simulink model "Modelo_UAV"  (R2017b)
settings: Solver=FixedStepAuto  StartTime=0.0  StopTime=6  FixedStep=1/10000  RelTol=1e-3
values from neighbouring files (symbols this model uses):
  Jcm_x = 7.5e3    (= 7500)    [UAV_parametros.m]
  Jcm_y = 7.5e3    (= 7500)    [UAV_parametros.m]
  Jcm_z = 14e3    (= 14000)    [UAV_parametros.m]
  M_t = 0.6    [UAV_parametros.m]
undefined symbols (not defined in the file or in its folder): sigbuilder_block
libraries: simulink x4
settings Model: Creator=JUANSEBASTIAN  LastModifiedBy=JUANSEBASTIAN
settings OptimizationCC: LifeSpan=inf
settings DebuggingCC: SFExecutionAtInitializationDiag=none
settings CodeAppCC: StateflowObjectComments=on

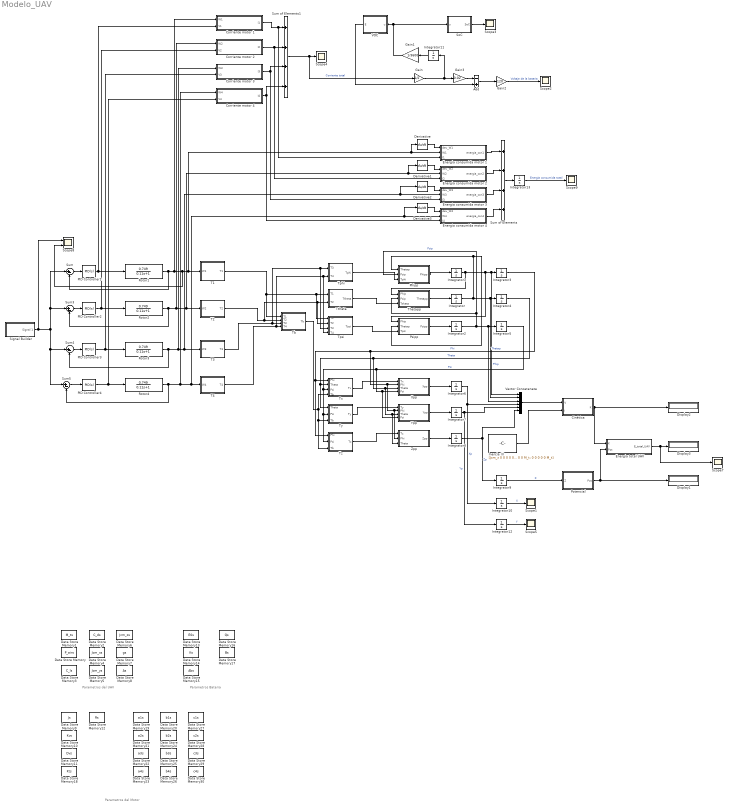
== system Modelo_UAV ==
  note: Parametros del UAV
  note: Parametros del Motor
  note: Parametros Bateria
  Add : Sum  Inputs=-+
  Cinética : MATLAB Function  TreatAsAtomicUnit=on
  Corriente motor 1 : MATLAB Function  TreatAsAtomicUnit=on
  Corriente motor 2 : MATLAB Function  TreatAsAtomicUnit=on
  Corriente motor 3 : MATLAB Function  TreatAsAtomicUnit=on
  Corriente motor 4 : MATLAB Function  TreatAsAtomicUnit=on
  Data Store Memory : DataStoreMemory  DataStoreName=P_airs  ReadBeforeWriteMsg=warning  WriteAfterWriteMsg=warning  WriteAfterReadMsg=warning  InitialValue=P_air  ShowAdditionalParam=off  OutDataTypeStr=double
      settings: LockScale=on
  Data Store Memory1 : DataStoreMemory  DataStoreName=M_ts  ReadBeforeWriteMsg=warning  WriteAfterWriteMsg=warning  WriteAfterReadMsg=warning  InitialValue=M_t  ShowAdditionalParam=off  OutDataTypeStr=double
      settings: LockScale=on
  Data Store Memory10 : DataStoreMemory  DataStoreName=Kvs  ReadBeforeWriteMsg=warning  WriteAfterWriteMsg=warning  WriteAfterReadMsg=warning  InitialValue=Kv  ShowAdditionalParam=off  OutDataTypeStr=double
      settings: LockScale=on
  Data Store Memory11 : DataStoreMemory  DataStoreName=Dvs  ReadBeforeWriteMsg=warning  WriteAfterWriteMsg=warning  WriteAfterReadMsg=warning  InitialValue=Dv  ShowAdditionalParam=off  OutDataTypeStr=double
      settings: LockScale=on
  Data Store Memory12 : DataStoreMemory  DataStoreName=Rs  ReadBeforeWriteMsg=warning  WriteAfterWriteMsg=warning  WriteAfterReadMsg=warning  InitialValue=R  ShowAdditionalParam=off  OutDataTypeStr=double
      settings: LockScale=on
  Data Store Memory13 : DataStoreMemory  DataStoreName=E0s  ReadBeforeWriteMsg=warning  WriteAfterWriteMsg=warning  WriteAfterReadMsg=warning  InitialValue=E0  ShowAdditionalParam=off  OutDataTypeStr=double
      settings: LockScale=on
  Data Store Memory14 : DataStoreMemory  DataStoreName=Ks  ReadBeforeWriteMsg=warning  WriteAfterWriteMsg=warning  WriteAfterReadMsg=warning  InitialValue=K  ShowAdditionalParam=off  OutDataTypeStr=double
      settings: LockScale=on
  Data Store Memory15 : DataStoreMemory  DataStoreName=Abs  ReadBeforeWriteMsg=warning  WriteAfterWriteMsg=warning  WriteAfterReadMsg=warning  InitialValue=Ab  ShowAdditionalParam=off  OutDataTypeStr=double
      settings: LockScale=on
  Data Store Memory16 : DataStoreMemory  DataStoreName=Qs  ReadBeforeWriteMsg=warning  WriteAfterWriteMsg=warning  WriteAfterReadMsg=warning  InitialValue=Q  ShowAdditionalParam=off  OutDataTypeStr=double
      settings: LockScale=on
  Data Store Memory17 : DataStoreMemory  DataStoreName=Bs  ReadBeforeWriteMsg=warning  WriteAfterWriteMsg=warning  WriteAfterReadMsg=warning  InitialValue=B  ShowAdditionalParam=off  OutDataTypeStr=double
      settings: LockScale=on
  Data Store Memory18 : DataStoreMemory  DataStoreName=Kts  ReadBeforeWriteMsg=warning  WriteAfterWriteMsg=warning  WriteAfterReadMsg=warning  InitialValue=Kt  ShowAdditionalParam=off  OutDataTypeStr=double
      settings: LockScale=on
  Data Store Memory19 : DataStoreMemory  DataStoreName=a1s  ReadBeforeWriteMsg=warning  WriteAfterWriteMsg=warning  WriteAfterReadMsg=warning  InitialValue=a1  ShowAdditionalParam=off  OutDataTypeStr=double
      settings: LockScale=on
  Data Store Memory2 : DataStoreMemory  DataStoreName=C_ds  ReadBeforeWriteMsg=warning  WriteAfterWriteMsg=warning  WriteAfterReadMsg=warning  InitialValue=C_d  ShowAdditionalParam=off  OutDataTypeStr=double
      settings: LockScale=on
  Data Store Memory20 : DataStoreMemory  DataStoreName=b1s  ReadBeforeWriteMsg=warning  WriteAfterWriteMsg=warning  WriteAfterReadMsg=warning  InitialValue=b1  ShowAdditionalParam=off  OutDataTypeStr=double
      settings: LockScale=on
  Data Store Memory21 : DataStoreMemory  DataStoreName=a2s  ReadBeforeWriteMsg=warning  WriteAfterWriteMsg=warning  WriteAfterReadMsg=warning  InitialValue=a2  ShowAdditionalParam=off  OutDataTypeStr=double
      settings: LockScale=on
  Data Store Memory22 : DataStoreMemory  DataStoreName=a3s  ReadBeforeWriteMsg=warning  WriteAfterWriteMsg=warning  WriteAfterReadMsg=warning  InitialValue=a3  ShowAdditionalParam=off  OutDataTypeStr=double
      settings: LockScale=on
  Data Store Memory23 : DataStoreMemory  DataStoreName=a4s  ReadBeforeWriteMsg=warning  WriteAfterWriteMsg=warning  WriteAfterReadMsg=warning  InitialValue=a4  ShowAdditionalParam=off  OutDataTypeStr=double
      settings: LockScale=on
  Data Store Memory24 : DataStoreMemory  DataStoreName=b2s  ReadBeforeWriteMsg=warning  WriteAfterWriteMsg=warning  WriteAfterReadMsg=warning  InitialValue=b2  ShowAdditionalParam=off  OutDataTypeStr=double
      settings: LockScale=on
  Data Store Memory25 : DataStoreMemory  DataStoreName=b3s  ReadBeforeWriteMsg=warning  WriteAfterWriteMsg=warning  WriteAfterReadMsg=warning  InitialValue=b3  ShowAdditionalParam=off  OutDataTypeStr=double
      settings: LockScale=on
  Data Store Memory26 : DataStoreMemory  DataStoreName=b4s  ReadBeforeWriteMsg=warning  WriteAfterWriteMsg=warning  WriteAfterReadMsg=warning  InitialValue=b4  ShowAdditionalParam=off  OutDataTypeStr=double
      settings: LockScale=on
  Data Store Memory27 : DataStoreMemory  DataStoreName=c1s  ReadBeforeWriteMsg=warning  WriteAfterWriteMsg=warning  WriteAfterReadMsg=warning  InitialValue=c1  ShowAdditionalParam=off  OutDataTypeStr=double
      settings: LockScale=on
  Data Store Memory28 : DataStoreMemory  DataStoreName=c2s  ReadBeforeWriteMsg=warning  WriteAfterWriteMsg=warning  WriteAfterReadMsg=warning  InitialValue=c2  ShowAdditionalParam=off  OutDataTypeStr=double
      settings: LockScale=on
  Data Store Memory29 : DataStoreMemory  DataStoreName=c3s  ReadBeforeWriteMsg=warning  WriteAfterWriteMsg=warning  WriteAfterReadMsg=warning  InitialValue=c3  ShowAdditionalParam=off  OutDataTypeStr=double
      settings: LockScale=on
  Data Store Memory3 : DataStoreMemory  DataStoreName=C_ls  ReadBeforeWriteMsg=warning  WriteAfterWriteMsg=warning  WriteAfterReadMsg=warning  InitialValue=C_l  ShowAdditionalParam=off  OutDataTypeStr=double
      settings: LockScale=on
  Data Store Memory30 : DataStoreMemory  DataStoreName=c4s  ReadBeforeWriteMsg=warning  WriteAfterWriteMsg=warning  WriteAfterReadMsg=warning  InitialValue=c4  ShowAdditionalParam=off  OutDataTypeStr=double
      settings: LockScale=on
  Data Store Memory4 : DataStoreMemory  DataStoreName=Jcm_xs  ReadBeforeWriteMsg=warning  WriteAfterWriteMsg=warning  WriteAfterReadMsg=warning  InitialValue=Jcm_x  ShowAdditionalParam=off  OutDataTypeStr=double
      settings: LockScale=on
  Data Store Memory5 : DataStoreMemory  DataStoreName=Jcm_ys  ReadBeforeWriteMsg=warning  WriteAfterWriteMsg=warning  WriteAfterReadMsg=warning  InitialValue=Jcm_y  ShowAdditionalParam=off  OutDataTypeStr=double
      settings: LockScale=on
  Data Store Memory6 : DataStoreMemory  DataStoreName=Jcm_zs  ReadBeforeWriteMsg=warning  WriteAfterWriteMsg=warning  WriteAfterReadMsg=warning  InitialValue=Jcm_z  ShowAdditionalParam=off  OutDataTypeStr=double
      settings: LockScale=on
  Data Store Memory7 : DataStoreMemory  DataStoreName=gs  ReadBeforeWriteMsg=warning  WriteAfterWriteMsg=warning  WriteAfterReadMsg=warning  InitialValue=g  ShowAdditionalParam=off  OutDataTypeStr=double
      settings: LockScale=on
  Data Store Memory8 : DataStoreMemory  DataStoreName=As  ReadBeforeWriteMsg=warning  WriteAfterWriteMsg=warning  WriteAfterReadMsg=warning  InitialValue=A  ShowAdditionalParam=off  OutDataTypeStr=double
      settings: LockScale=on
  Data Store Memory9 : DataStoreMemory  DataStoreName=Js  ReadBeforeWriteMsg=warning  WriteAfterWriteMsg=warning  WriteAfterReadMsg=warning  InitialValue=J  ShowAdditionalParam=off  OutDataTypeStr=double
      settings: LockScale=on
  Derivative{,1..3} (4 alike) : Derivative
  Display1 : Display
  Display2 : Display
  Display3 : Display
  Energia consumida motor 1 : MATLAB Function  TreatAsAtomicUnit=on
  "Energia consumida motor 2 " : MATLAB Function  TreatAsAtomicUnit=on
  Energia consumida motor 3 : MATLAB Function  TreatAsAtomicUnit=on
  Energia consumida motor 4 : MATLAB Function  TreatAsAtomicUnit=on
  Energia total UAV : MATLAB Function  TreatAsAtomicUnit=on
  Gain : Gain  Gain=1/2
  Gain1 : Gain  Gain=1/3600
  Gain2 : Gain  Gain=120
  Gain3 : Gain  Gain=0.02
  Inercia (I) : Constant  Value=[Jcm_x 0 0 0 0 0; 0 Jcm_y 0 0 0 0; 0 0 Jcm_z 0 0 0; 0 0 0 M_t 0 0; 0 0 0 0 0 M_t; 0 0 0 0 0 M_t]
  Integrator{,1..12} (13 alike) : Integrator
  Integrator13 : Integrator  UpperSaturationLimit=6  LowerSaturationLimit=0
  PID Controller{1..4} (4 alike) : simulink/Continuous/PID Controller  Controller=PID  TimeDomain=Continuous-time  SampleTime=-1  IntegratorMethod=Forward Euler  FilterMethod=Forward Euler  Form=Parallel  UseFilter=on  ControllerParametersSource=internal  P=1.58016  I=41.7167  D=-65.339e-3  N=200  InitialConditionSource=internal  InitialConditionForIntegrator=0  InitialConditionForFilter=0  ExternalReset=none  LimitOutput=off  UpperSaturationLimit=inf  LowerSaturationLimit=-inf  LinearizeAsGain=on  AntiWindupMode=none  Kb=1  TrackingMode=off  Kt=1  PParamMin=[]  PParamMax=[]  IParamMin=[]  IParamMax=[]  DParamMin=[]  DParamMax=[]  NParamMin=[]  NParamMax=[]  KbParamMin=[]  KbParamMax=[]  KtParamMin=[]  KtParamMax=[]  POutMin=[]  POutMax=[]  IOutMin=[]  IOutMax=[]  DOutMin=[]  DOutMax=[]  NOutMin=[]  NOutMax=[]  KbOutMin=[]  KbOutMax=[]  KtOutMin=[]  KtOutMax=[]  IntegratorOutMin=[]  IntegratorOutMax=[]  FilterOutMin=[]  FilterOutMax=[]  SumOutMin=[]  SumOutMax=[]  SumI1OutMin=[]  SumI1OutMax=[]  SumI2OutMin=[]  SumI2OutMax=[]  SumI3OutMin=[]  SumI3OutMax=[]  SumDOutMin=[]  SumDOutMax=[]  SaturationOutMin=[]  SaturationOutMax=[]  IntegratorContinuousStateAttributes=''  IntegratorStateMustResolveToSignalObject=off  IntegratorRTWStateStorageClass=Auto  FilterContinuousStateAttributes=''  FilterStateMustResolveToSignalObject=off  FilterRTWStateStorageClass=Auto  DifferentiatorICPrevScaledInput=0  DifferentiatorOutMin=[]  DifferentiatorOutMax=[]  InitialConditionSetting=State (most efficient)  FilterDiffOutCoefMin=[]  FilterDiffOutCoefMax=[]  SumDenOutMin=[]  SumDenOutMax=[]  SumNumOutMin=[]  SumNumOutMax=[]  ReciprocalOutMin=[]  ReciprocalOutMax=[]  DivideOutMin=[]  DivideOutMax=[]  TunerSelectOption=Transfer Function Based (PID Tuner App)
  Phipp : MATLAB Function  TreatAsAtomicUnit=on
  Potencial : MATLAB Function  TreatAsAtomicUnit=on
  Psipp : MATLAB Function  TreatAsAtomicUnit=on
  Rotor{1..4} (4 alike) : TransferFcn  Numerator=[0.749]  Denominator=[0.11 1]
  Scope{1..5,7,9} (7 alike) : Scope
  Scope8 : Scope  NumInputPorts=2
  Signal Builder : Subsystem  Tag=STV Subsys  LoadFcn=sigbuilder_block('load',[6 6 1012.5 506.25 ]);  StartFcn=sigbuilder_block('start');  StopFcn=sigbuilder_block('stop');  ClipboardFcn=sigbuilder_block('clipboard');  mask(Sigbuilder block){tuvar=[0:10]}
      mask help: Simulink:masks:SigbuilderBlock_MD
      mask init:
      | if ~strcmp(get_param(bdroot(gcbh),'SimulationStatus'),'stopped') tuvar = sigbuilder_block('maskInit'); end
      settings: CopyFcn=sigbuilder_block('copy');  DeleteFcn=sigbuilder_block('delete');  ModelCloseFcn=sigbuilder_block('modelClose');  PreSaveFcn=sigbuilder_block('preSave');  PauseFcn=sigbuilder_block('pause');  ContinueFcn=sigbuilder_block('continue');  NameChangeFcn=sigbuilder_block('namechange');  OpenFcn=sigbuilder_block('open',[6 6 1012.5 506.25 ]);  CloseFcn=sigbuilder_block('close');
      mask Display: plot(0, 0, 100, 100,[2, 2, 32, 32, 2], [68, 8, 8, 68, 68],[32, 2], [38, 38], [32, 19, 2],[53, 60, 44], [32, 17, 17, 2],[16, 16, 31, 31]);txt = getActiveGroup(gcbh);text(2, 100, txt,'verticalAlignment', 'top');
  "SoC " : MATLAB Function  TreatAsAtomicUnit=on
  Sum{,3..5} (4 alike) : Sum  Inputs=|+-
  Sum of Elements : Sum  Inputs=++++
  Sum of Elements1 : Sum  Inputs=++++
  T1 : MATLAB Function  TreatAsAtomicUnit=on
  T2 : MATLAB Function  TreatAsAtomicUnit=on
  T3 : MATLAB Function  TreatAsAtomicUnit=on
  T4 : MATLAB Function  TreatAsAtomicUnit=on
  Tb : MATLAB Function  TreatAsAtomicUnit=on
  Thetapp : MATLAB Function  TreatAsAtomicUnit=on
  Tphi : MATLAB Function  TreatAsAtomicUnit=on
  Tpsi : MATLAB Function  TreatAsAtomicUnit=on
  Ttheta : MATLAB Function  TreatAsAtomicUnit=on
  Tx : MATLAB Function  TreatAsAtomicUnit=on
  Ty : MATLAB Function  TreatAsAtomicUnit=on
  Tz : MATLAB Function  TreatAsAtomicUnit=on
  VOC : MATLAB Function  TreatAsAtomicUnit=on
  Vector Concatenate : Concatenate  NumInputs=6
  Xpp : MATLAB Function  TreatAsAtomicUnit=on
  Ypp : MATLAB Function  TreatAsAtomicUnit=on
  Zpp : MATLAB Function  TreatAsAtomicUnit=on
  wires:
  Sum/1 -> PID Controller1/1
  PID Controller1/1 -> Corriente motor 1/2(V1), Rotor1/1
  Rotor1/1 -> Corriente motor 1/1(W1), Scope8/2, Energia consumida motor 1/2(W1), Derivative/1, T1/1(W1), Sum/2
  Sum3/1 -> PID Controller2/1
  Rotor2/1 -> Corriente motor 2/1(W2), Derivative1/1, "Energia consumida motor 2 "/2(W2), T2/1(W2), Sum3/2
  PID Controller2/1 -> Corriente motor 2/2(V2), Rotor2/1
  Sum4/1 -> PID Controller3/1
  Rotor3/1 -> Corriente motor 3/1(W3), Derivative2/1, Energia consumida motor 3/2(W3), T3/1(W3), Sum4/2
  PID Controller3/1 -> Corriente motor 3/2(V3), Rotor3/1
  Sum5/1 -> PID Controller4/1
  Rotor4/1 -> Derivative3/1, Energia consumida motor 4/2(W4), T4/1(W4), Corriente motor 4/1(W4), Sum5/2
  PID Controller4/1 -> Corriente motor 4/2(V4), Rotor4/1
  Signal Builder/1(Signal 1) -> Scope8/1, Sum4/1, Sum5/1, Sum/1, Sum3/1
  T1/1(T1) -> Tb/1(T1), Tpsi/1(T1), Ttheta/1(T1)
  T2/1(T2) -> Tpsi/2(T2), Ttheta/2(T2), Tb/2(T2)
  T3/1(T3) -> Tpsi/3(T3), Tphi/1(T3), Tb/3(T3)
  T4/1(T4) -> Tpsi/4(T4), Tphi/2(T4), Tb/4(T4)
  Tb/1(Tb) -> Tz/3(Tb), Ty/3(Tb), Tx/4(Tb)
  Tphi/1(Tphi) -> Phipp/3(Tphi)
  Thetapp/1(Thetapp) -> Integrator/1
  Integrator/1 -> Vector Concatenate/2, Integrator4/1, Phipp/1(Thetap), Psipp/2(Thetap)  "Thetap"
  Ttheta/1(Ttheta) -> Thetapp/3(Ttheta)
  Phipp/1(Phipp) -> Integrator1/1
  Integrator1/1 -> Vector Concatenate/1, Integrator3/1, Psipp/1(Phip), Thetapp/1(Phip)  "Phip"
  Psipp/1(Psipp) -> Integrator2/1
  Integrator2/1 -> Vector Concatenate/3, Integrator5/1, Thetapp/2(Psip), Phipp/2(Psip)  "Psip"
  Tpsi/1(Tpsi) -> Psipp/3(Tpsi)
  Integrator3/1 -> Tx/1(Phi), Tz/1(Phi), Xpp/2(Phi), Zpp/2(Phi), Ypp/2(Phi)  "Phi"
  Integrator4/1 -> Xpp/3(Theta), Zpp/3(Theta), Ypp/3(Theta), Ty/1(Theta), Tx/2(Theta)  "Theta"
  Integrator5/1 -> Xpp/4(Psi), Ypp/4(Psi), Tz/2(Psi), Ty/2(Psi), Tx/3(Psi)  "Psi"
  Tx/1(Tx) -> Xpp/1(Tx)
  Ty/1(Ty) -> Ypp/1(Ty)
  Tz/1(Tz) -> Zpp/1(Tz)
  Ypp/1(Ypp) -> Integrator7/1
  Zpp/1(Zpp) -> Integrator8/1
  Xpp/1(Xpp) -> Integrator6/1
  Vector Concatenate/1 -> Cinética/1(V)
  Inercia (I)/1 -> Cinética/2(I)
  Cinética/1(K) -> Energia total UAV/1(K), Display2/1
  Integrator6/1 -> Vector Concatenate/4, Integrator10/1  "Xp"
  Integrator7/1 -> Integrator12/1, Vector Concatenate/5  "Yp"
  Integrator8/1 -> Integrator9/1, Vector Concatenate/6  "Zp"
  Integrator9/1 -> Potencial/1(Z)  "Z"
  Potencial/1(Pot) -> Energia total UAV/2(Pot), Display1/1
  Energia total UAV/1(E_total_UAV) -> Scope7/1, Display3/1
  Integrator10/1 -> Scope1/1  "X"
  Gain3/1 -> Add/1
  Gain2/1 -> Scope2/1  "Voltaje de la bateria"
  Integrator11/1 -> Gain1/1
  Gain1/1 -> "SoC "/1(u), VOC/1(u)
  Add/1 -> Gain2/1
  "SoC "/1(SoC) -> Scope3/1
  Gain/1 -> Gain3/1, Integrator11/1
  VOC/1(E) -> Add/2
  Integrator12/1 -> Scope5/1  "Y"
  Derivative/1 -> Energia consumida motor 1/1(dev_W1)
  Derivative1/1 -> "Energia consumida motor 2 "/1(dev_W2)
  Derivative2/1 -> Energia consumida motor 3/1(dev_W3)
  Derivative3/1 -> Energia consumida motor 4/1(dev_W4)
  Sum of Elements/1 -> Integrator13/1
  Integrator13/1 -> Scope9/1  "Energia consumida total"
  Energia consumida motor 1/1(energia_con1) -> Sum of Elements/1
  Energia consumida motor 3/1(energia_con3) -> Sum of Elements/3
  Energia consumida motor 4/1(energia_con4) -> Sum of Elements/4
  Sum of Elements1/1 -> Gain/1, Scope4/1  "Corriente total"
  Corriente motor 1/1(I1) -> Sum of Elements1/1, Energia consumida motor 1/3(I1)
  Corriente motor 2/1(I2) -> Sum of Elements1/2, "Energia consumida motor 2 "/3(I2)
  Corriente motor 3/1(I3) -> Energia consumida motor 3/3(I3), Sum of Elements1/3
  Corriente motor 4/1(I4) -> Energia consumida motor 4/3(I4), Sum of Elements1/4
  "Energia consumida motor 2 "/1(energia_con2) -> Sum of Elements/2

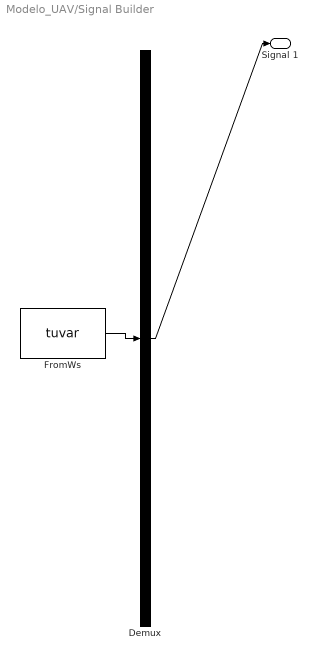
== system Modelo_UAV/Signal Builder ==
  Demux : Demux  Tag=STV Demux  Outputs=1
  FromWs : FromWorkspace  Tag=STV FromWs  VariableName=tuvar  SampleTime=0
      SigBuilderData=|
      | common.afterFinalStr = 'Extrapolate'
      | common.sampleTime = 0
      | dataSet.timeRange = [0 6]
      | dataSet.name = 'Group 1'
      | sbobj.Groups.Name = 'Group 1'
      | sbobj.Groups.Signals.Name = 'Signal 1'
      | sbobj.Groups.Signals.XData = [0 2 4 6]
      | sbobj.Groups.Signals.YData = [0 3000 3000 0]
      | sbobj.Groups.TimeRange = [0 6]
  Signal 1 : Outport  Tag=STV Outport
  wires:
  FromWs/1 -> Demux/1
  Demux/1 -> Signal 1/1

== matlab function Modelo_UAV/T2 ==
  settings: updateMethod=DISCRETE
  data: W2 input; T2 output; P_airs data_store_memory; C_ls data_store_memory; C_ds data_store_memory; As data_store_memory
function T2 = fcn(W2)
global P_airs;
global C_ls;
global C_ds;
global As;
T2 = (1/2)*P_airs*(W2^2)*As*(C_ls+C_ds);

== matlab function Modelo_UAV/T1 ==
  settings: updateMethod=DISCRETE
  data: W1 input; T1 output; P_airs data_store_memory; C_ls data_store_memory; C_ds data_store_memory; As data_store_memory
function T1 = fcn(W1)
global P_airs;
global C_ls;
global C_ds;
global As;
T1 = (1/2)*P_airs*(W1^2)*As*(C_ls+C_ds);

== matlab function Modelo_UAV/T4 ==
  settings: updateMethod=DISCRETE
  data: W4 input; T4 output; P_airs data_store_memory; C_ls data_store_memory; C_ds data_store_memory; As data_store_memory
function T4 = fcn(W4)
global P_airs;
global C_ls;
global C_ds;
global As;
T4 = (1/2)*P_airs*(W4^2)*As*(C_ls+C_ds);

== matlab function Modelo_UAV/T3 ==
  settings: updateMethod=DISCRETE
  data: W3 input; T3 output; P_airs data_store_memory; C_ls data_store_memory; C_ds data_store_memory; As data_store_memory
function T3 = fcn(W3)
global P_airs;
global C_ls;
global C_ds;
global As;
T3 = (1/2)*P_airs*(W3^2)*As*(C_ls+C_ds);

== matlab function Modelo_UAV/Tb ==
  data: T1 input; Tb output; T2 input; T3 input; T4 input
function Tb = fcn(T1,T2,T3,T4)

Tb = (T1+T2+T3+T4);

== matlab function Modelo_UAV/Tphi ==
  data: Tphi output; T3 input; T4 input
function Tphi = fcn(T3,T4)

Tphi = 0.15*(T4-T3);

== matlab function Modelo_UAV/Ttheta ==
  data: Ttheta output; T1 input; T2 input
function Ttheta = fcn(T1,T2)

Ttheta = 0.15*(T1-T2);

== matlab function Modelo_UAV/Tpsi ==
  data: Tpsi output; T1 input; T2 input; T3 input; T4 input
function Tpsi = fcn(T1,T2,T3,T4)

Tpsi = 0.15*(T3+T4-T1-T2);

== matlab function Modelo_UAV/Phipp ==
  settings: updateMethod=DISCRETE
  data: Phipp output; Thetap input; Psip input; Tphi input; Jcm_xs data_store_memory; Jcm_ys data_store_memory; Jcm_zs data_store_memory
function Phipp = fcn(Thetap,Psip,Tphi)
global Jcm_xs;
global Jcm_ys;
global Jcm_zs;
Phipp = ((((Jcm_ys)-(Jcm_zs))/(Jcm_xs))*Thetap*Psip)+((1/(Jcm_xs))*Tphi);

== matlab function Modelo_UAV/Thetapp ==
  settings: updateMethod=DISCRETE
  data: Thetapp output; Phip input; Psip input; Ttheta input; Jcm_xs data_store_memory; Jcm_ys data_store_memory; Jcm_zs data_store_memory
function Thetapp = fcn(Phip,Psip,Ttheta)
global Jcm_xs;
global Jcm_ys;
global Jcm_zs;
Thetapp = ((((Jcm_ys)-(Jcm_zs))/(Jcm_xs))*Phip*Psip)+((1/(Jcm_ys))*Ttheta);

== matlab function Modelo_UAV/Psipp ==
  settings: updateMethod=DISCRETE
  data: Psipp output; Phip input; Thetap input; Tpsi input; Jcm_xs data_store_memory; Jcm_ys data_store_memory; Jcm_zs data_store_memory
function Psipp = fcn(Phip,Thetap,Tpsi)
global Jcm_xs;
global Jcm_ys;
global Jcm_zs;
Psipp = ((((Jcm_xs)-(Jcm_ys))/(Jcm_zs))*Phip*Thetap)+((1/(Jcm_zs))*Tpsi);

== matlab function Modelo_UAV/Tx ==
  data: Phi input; Theta input; Tx output; Psi input; Tb input
function Tx = fcn(Phi,Theta,Psi,Tb)

Tx = ((sin(Psi)*sin(Theta))+(cos(Psi)*sin(Theta)*cos(Phi)))*Tb;

== matlab function Modelo_UAV/Ty ==
  data: Theta input; Ty output; Psi input; Tb input
function Ty = fcn(Theta,Psi,Tb)

Ty = ((-cos(Psi)*sin(Theta))+(sin(Psi)*sin(Theta)*cos(Theta)))*Tb;

== matlab function Modelo_UAV/Tz ==
  data: Phi input; Tz output; Psi input; Tb input
function Tz = fcn(Phi,Psi,Tb)

Tz = ((-cos(Psi)*cos(Phi)))*Tb;

== matlab function Modelo_UAV/Xpp ==
  settings: updateMethod=DISCRETE
  data: Xpp output; Tx input; Phi input; Theta input; Psi input; M_ts data_store_memory
function Xpp = fcn(Tx,Phi,Theta,Psi)
global M_ts;
Xpp = Tx*(((cos(Phi)*sin(Theta)*cos(Psi))+(sin(Phi)+sin(Psi)))/M_ts);

== matlab function Modelo_UAV/Ypp ==
  settings: updateMethod=DISCRETE
  data: Ypp output; Ty input; Phi input; Theta input; Psi input; M_ts data_store_memory
function Ypp = fcn(Ty,Phi,Theta,Psi)
global M_ts;
Ypp = Ty*(((cos(Phi)*sin(Theta)*cos(Psi))-(sin(Phi)+cos(Psi)))/M_ts);

== matlab function Modelo_UAV/Zpp ==
  settings: updateMethod=DISCRETE
  data: Zpp output; Tz input; Phi input; Theta input; M_ts data_store_memory; gs data_store_memory
function Zpp = fcn(Tz,Phi,Theta)
global M_ts;
global gs;
Zpp = Tz*(((cos(Phi)*cos(Theta))-(gs))/M_ts);

== matlab function Modelo_UAV/Cinética ==
  data: K output; V input; I input
function K = fcn(V,I)
V_trans=transpose(V);
K = (1/2)*V_trans*I*V;

== matlab function Modelo_UAV/Potencial ==
  data: Pot output; Z input
function Pot = fcn(Z)
P = 0.6*9.81*Z;
Pot=abs(P)

== matlab function Modelo_UAV/Energia total UAV ==
  data: E_total_UAV output; K input; Pot input
function E_total_UAV = fcn(K,Pot)

E_total_UAV = K+Pot;

== matlab function Modelo_UAV/VOC ==
  settings: updateMethod=DISCRETE
  data: E output; u input; E0s data_store_memory; Ks data_store_memory; Abs data_store_memory; Qs data_store_memory; Bs data_store_memory
function E = fcn(u)
global E0s;
global Ks;
global Abs;
global Qs;
global Bs;

E=E0s-Ks*(Qs/(Qs-u(1)))+Abs*exp(-Bs*u(1));

== matlab function Modelo_UAV/SoC  ==
  settings: updateMethod=DISCRETE
  data: u input; SoC output; Qs data_store_memory
function SoC = fcn(u)
global Qs; %Amperios hora
%SoC = 100*(1-(u/Qs));
SoC = 100*(1-(u/Qs));

== matlab function Modelo_UAV/Corriente motor 1 ==
  settings: updateMethod=DISCRETE
  data: W1 input; V1 input; I1 output; Rs data_store_memory; Kvs data_store_memory
function I1 = fcn(W1, V1)
global Rs;
global Kvs;
COR1=(V1-(W1/Kvs))/Rs;
I1=abs(COR1)

== matlab function Modelo_UAV/Corriente motor 2 ==
  settings: updateMethod=DISCRETE
  data: W2 input; V2 input; I2 output; Rs data_store_memory; Kvs data_store_memory
function I2 = fcn(W2, V2)
global Rs;
global Kvs;
COR2=(V2-(W2/Kvs))/Rs;
I2=abs(COR2)

== matlab function Modelo_UAV/Corriente motor 3 ==
  settings: updateMethod=DISCRETE
  data: W3 input; V3 input; I3 output; Rs data_store_memory; Kvs data_store_memory
function I3 = fcn(W3, V3)
global Rs;
global Kvs;
COR3=(V3-(W3/Kvs))/Rs;
I3=abs(COR3)

== matlab function Modelo_UAV/Corriente motor 4 ==
  settings: updateMethod=DISCRETE
  data: W4 input; V4 input; I4 output; Rs data_store_memory; Kvs data_store_memory
function I4 = fcn(W4, V4)
global Rs;
global Kvs;
COR4=(V4-(W4/Kvs))/Rs;
I4=abs(COR4)

== matlab function Modelo_UAV/Energia consumida motor 1 ==
  settings: updateMethod=DISCRETE
  data: dev_W1 input; energia_con1 output; W1 input; Js data_store_memory; Dvs data_store_memory; I1 input; Kts data_store_memory; C_ds data_store_memory; a1s data_store_memory; a2s data_store_memory; a3s data_store_memory; a4s data_store_memory; b1s data_store_memory; b2s data_store_memory; b3s data_store_memory; b4s data_store_memory; c1s data_store_memory; c2s data_store_memory; c3s data_store_memory; c4s data_store_memory
function energia_con1 = fcn(dev_W1, W1, I1)
global Js;
global Dvs;
global Kts;
global C_ds;
global a1s;
global a2s;
global a3s;
global a4s;
global b1s;
global b2s;
global b3s;
global b4s;
global c1s;
global c2s;
global c3s;
global c4s;

a=(a1s*(W1^2))+(b1s*W1)+c1s;
b=(a2s*(W1^2))+(b2s*W1)+c2s;
c=(a3s*(W1^2))+(b3s*W1)+c3s;
d=(a4s*(W1^2))+(b4s*W1)+c4s;

Tor=I1*Kts;
fr=(a*(Tor^3))+(b*(Tor^2))+(c*Tor)+d;
energia_con1=(((Js*dev_W1)+(C_ds*(W1^2))+(Dvs*W1))*W1)/fr;

== matlab function Modelo_UAV/Energia consumida motor 2  ==
  settings: updateMethod=DISCRETE
  data: dev_W2 input; energia_con2 output; W2 input; Js data_store_memory; Dvs data_store_memory; I2 input; Kts data_store_memory; C_ds data_store_memory; a1s data_store_memory; a2s data_store_memory; a3s data_store_memory; a4s data_store_memory; b1s data_store_memory; b2s data_store_memory; b3s data_store_memory; b4s data_store_memory; c1s data_store_memory; c2s data_store_memory; c3s data_store_memory; c4s data_store_memory
function energia_con2 = fcn(dev_W2, W2, I2)
global Js;
global Dvs;
global Kts;
global C_ds;
global a1s;
global a2s;
global a3s;
global a4s;
global b1s;
global b2s;
global b3s;
global b4s;
global c1s;
global c2s;
global c3s;
global c4s;

a=(a1s*(W2^2))+(b1s*W2)+c1s;
b=(a2s*(W2^2))+(b2s*W2)+c2s;
c=(a3s*(W2^2))+(b3s*W2)+c3s;
d=(a4s*(W2^2))+(b4s*W2)+c4s;

Tor=I2*Kts;
fr=(a*Tor^3)+(b*Tor^2)+(c*Tor)+d;
energia_con2=(((Js*dev_W2)+(C_ds*(W2^2))+(Dvs*W2))*W2)/fr;

== matlab function Modelo_UAV/Energia consumida motor 3 ==
  settings: updateMethod=DISCRETE
  data: dev_W3 input; energia_con3 output; W3 input; Js data_store_memory; Dvs data_store_memory; I3 input; Kts data_store_memory; C_ds data_store_memory; a1s data_store_memory; a2s data_store_memory; a3s data_store_memory; a4s data_store_memory; b1s data_store_memory; b2s data_store_memory; b3s data_store_memory; b4s data_store_memory; c1s data_store_memory; c2s data_store_memory; c3s data_store_memory; c4s data_store_memory
function energia_con3 = fcn(dev_W3, W3, I3)
global Js;
global Dvs;
global Kts;
global C_ds;
global a1s;
global a2s;
global a3s;
global a4s;
global b1s;
global b2s;
global b3s;
global b4s;
global c1s;
global c2s;
global c3s;
global c4s;

a=(a1s*(W3^2))+(b1s*W3)+c1s;
b=(a2s*(W3^2))+(b2s*W3)+c2s;
c=(a3s*(W3^2))+(b3s*W3)+c3s;
d=(a4s*(W3^2))+(b4s*W3)+c4s;

Tor=I3*Kts;
fr=(a*Tor^3)+(b*Tor^2)+(c*Tor)+d;
energia_con3=(((Js*dev_W3)+(C_ds*(W3^2))+(Dvs*W3))*W3)/fr;

== matlab function Modelo_UAV/Energia consumida motor 4 ==
  settings: updateMethod=DISCRETE
  data: dev_W4 input; energia_con4 output; W4 input; Js data_store_memory; Dvs data_store_memory; I4 input; Kts data_store_memory; C_ds data_store_memory; a1s data_store_memory; a2s data_store_memory; a3s data_store_memory; a4s data_store_memory; b1s data_store_memory; b2s data_store_memory; b3s data_store_memory; b4s data_store_memory; c1s data_store_memory; c2s data_store_memory; c3s data_store_memory; c4s data_store_memory
function energia_con4 = fcn(dev_W4, W4, I4)
global Js;
global Dvs;
global Kts;
global C_ds;
global a1s;
global a2s;
global a3s;
global a4s;
global b1s;
global b2s;
global b3s;
global b4s;
global c1s;
global c2s;
global c3s;
global c4s;

a=(a1s*(W4^2))+(b1s*W4)+c1s;
b=(a2s*(W4^2))+(b2s*W4)+c2s;
c=(a3s*(W4^2))+(b3s*W4)+c3s;
d=(a4s*(W4^2))+(b4s*W4)+c4s;

Tor=I4*Kts;
fr=(a*Tor^3)+(b*Tor^2)+(c*Tor)+d;
energia_con4=(((Js*dev_W4)+(C_ds*(W4^2))+(Dvs*W4))*W4)/fr;
